simulink model "Example_Simulation"  (R2023b)
settings: Solver=FixedStepAuto  StartTime=0.0  StopTime=50  FixedStep=0.01  RelTol=1e-3
values from neighbouring files (symbols this model uses):
  A1 = [-1 x2min; 0 -1]    [Example_Code.m]
  A2 = [-1 x2max; 0 -1]    [Example_Code.m]
  B = [0 1].'    [Example_Code.m]
  x2max = 0.3    [Example_Code.m]
  x2min = 0.1    [Example_Code.m]
undefined symbols (not defined in the file or in its folder): adis1, adis2, bdis1, bdis2
libraries: simulink x1
settings Model: Creator=adria  LastModifiedBy=adria

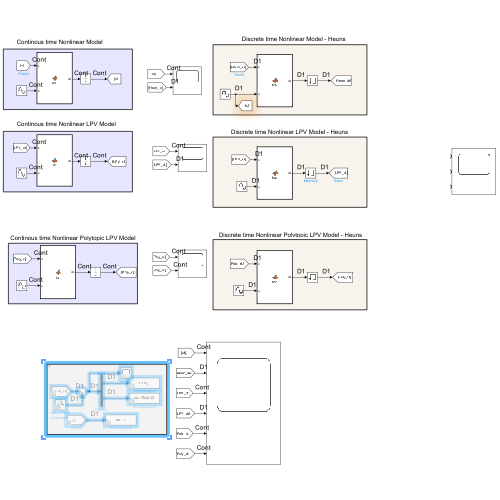
[thumbnail: Simulink's stored preview of the top-level diagram]
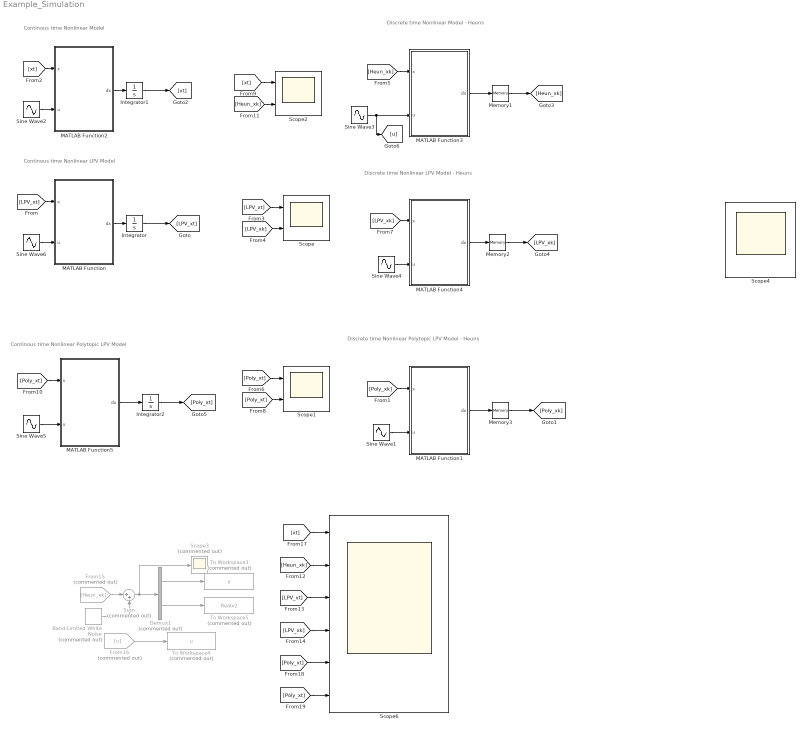
== system Example_Simulation ==
  note: Continous time Nonlinear LPV Model
  note: Continous time Nonlinear Model
  note: Discrete time Nonlinear Model - Heuns
  note: Discrete time Nonlinear LPV Model - Heuns
  note: Discrete time Nonlinear Polytopic LPV Model - Heuns
  note: Continous time Nonlinear Polytopic LPV Model
  Band-Limited White Noise : simulink/Sources/Band-Limited White Noise  Commented=on  Cov=[0.000001]  Ts=0.01  seed=[23341]
  Demux1 : Demux  Commented=on  Outputs=2
  From15 : From  Commented=on  GotoTag=Heun_xk
  From16 : From  Commented=on  GotoTag=u
  Integrator : Integrator  InitialCondition=[0 0.2].'
  Integrator1 : Integrator  InitialCondition=[0 0.2].'
  Integrator2 : Integrator  InitialCondition=[0 0.2].'
  MATLAB Function : MATLAB Function  TreatAsAtomicUnit=on
  MATLAB Function1 : MATLAB Function  TreatAsAtomicUnit=on
  MATLAB Function2 : MATLAB Function  TreatAsAtomicUnit=on
  MATLAB Function3 : MATLAB Function  TreatAsAtomicUnit=on
  MATLAB Function4 : MATLAB Function  TreatAsAtomicUnit=on
  MATLAB Function5 : MATLAB Function  TreatAsAtomicUnit=on
  Memory1 : Memory  InitialCondition=[0 0.2].'
  Memory2 : Memory  InitialCondition=[0 0.2].'
  Memory3 : Memory  InitialCondition=[0 0.2].'
  Scope : Scope  NumInputPorts=2
  Scope1 : Scope  NumInputPorts=2
  Scope2 : Scope  NumInputPorts=2
  Scope3 : Scope  Commented=on
  Scope4 : Scope  NumInputPorts=3
  Scope6 : Scope  NumInputPorts=6
  Sine Wave1 : Sin  Amplitude=0.1  Bias=0.2  Frequency=0.16  SampleTime=0.01
  Sine Wave2 : Sin  Amplitude=0.1  Bias=0.2  Frequency=0.16  SampleTime=0
  Sine Wave3 : Sin  Amplitude=0.1  Bias=0.2  Frequency=0.16  SampleTime=0.01
  Sine Wave4 : Sin  Amplitude=0.1  Bias=0.2  Frequency=0.16  SampleTime=0.01
  Sine Wave5 : Sin  Amplitude=0.1  Bias=0.2  Frequency=0.16  SampleTime=0
  Sine Wave6 : Sin  Amplitude=0.1  Bias=0.2  Frequency=0.16  SampleTime=0
  Sum : Sum  Commented=on  Inputs=|++
  To Workspace3 : ToWorkspace  Commented=on  VariableName=y  SaveFormat=Structure  SampleTime=-1
  To Workspace4 : ToWorkspace  Commented=on  VariableName=u  SaveFormat=Structure  SampleTime=-1
  To Workspace5 : ToWorkspace  Commented=on  VariableName=Realx2  SaveFormat=Structure  SampleTime=-1
  wires:
  MATLAB Function/1(dx) -> Integrator/1
  Integrator/1 -> [LPV_xt]
  Sine Wave6/1 -> MATLAB Function/2(u)
  [LPV_xt] -> MATLAB Function/1(x)
  [xt] -> MATLAB Function2/1(x)
  MATLAB Function2/1(dx) -> Integrator1/1
  Integrator1/1 -> [xt]
  Sine Wave2/1 -> MATLAB Function2/2(u)
  Memory1/1 -> [Heun_xk]
  Sine Wave3/1 -> [u], MATLAB Function3/2(u)
  [Heun_xk] -> MATLAB Function3/1(x)
  MATLAB Function3/1(dx) -> Memory1/1
  Sine Wave4/1 -> MATLAB Function4/2(u)
  MATLAB Function4/1(dx) -> Memory2/1
  [LPV_xk] -> MATLAB Function4/1(x)
  Memory2/1 -> [LPV_xk]
  Memory3/1 -> [Poly_xk]
  MATLAB Function1/1(dx) -> Memory3/1
  [Poly_xk] -> MATLAB Function1/1(x)
  Sine Wave1/1 -> MATLAB Function1/2(u)
  [Poly_xt] -> MATLAB Function5/1(x)
  Integrator2/1 -> [Poly_xt]
  MATLAB Function5/1(dx) -> Integrator2/1
  Sine Wave5/1 -> MATLAB Function5/2(u)
  [LPV_xt] -> Scope/1
  [LPV_xk] -> Scope/2
  [Poly_xt] -> Scope1/2
  [Poly_xt] -> Scope1/1
  [Heun_xk] -> Scope2/2
  [xt] -> Scope2/1
  [LPV_xk] -> Scope6/4
  [LPV_xt] -> Scope6/3
  [xt] -> Scope6/1
  [Heun_xk] -> Scope6/2
  [Poly_xt] -> Scope6/6
  [Poly_xt] -> Scope6/5
  Demux1/2 -> To Workspace5/1
  Demux1/1 -> To Workspace3/1
  From16/1 -> To Workspace4/1
  From15/1 -> Sum/1
  Band-Limited White Noise/1 -> Sum/2
  Sum/1 -> Scope3/1, Demux1/1

== matlab function Example_Simulation/MATLAB Function1 ==
  data: x input; u input; dx output; bdis1 parameter; adis2 parameter; adis1 parameter; bdis2 parameter; x2max parameter; x2min parameter
function dx  = fcn(x,u, bdis1, adis2, adis1, bdis2,x2max, x2min)


SchedulingMin = (x2max-x(2))/(x2max-x2min);
SchedulingMax = (1-SchedulingMin);

X = [x(1);x(2)];

dx = SchedulingMin*(adis1*X+bdis1*u) + SchedulingMax*(adis2*X+bdis2*u);

== matlab function Example_Simulation/MATLAB Function ==
  data: x input; dx output; u input
function dx = fcn(x,u)

X = [x(1);x(2)];
dx = [-1 x(2); 0 -1]*X+[0 1].'*u;

== matlab function Example_Simulation/MATLAB Function2 ==
  data: x input; dx output; u input
function dx = fcn(x,u)

dx1 = -x(1)+x(2)^2;
dx2 = -x(2)+u;
dx = [dx1;dx2];

== matlab function Example_Simulation/MATLAB Function3 ==
  data: x input; dx output; u input
function dx  = fcn(x,u)

dt = 0.01;
x1Predict = (-x(1)+x(2)^2)*dt+x(1);
x2Predict = (-x(2)+u)*dt+x(2);

T1 = -x(1)+x(2)^2;
N1 = -x1Predict+x2Predict^2;

T2 = -x(2)+u;
N2 = -x2Predict+u;

dx1 = x(1)+(dt/2)*(T1+N1);
dx2 = x(2)+(dt/2)*(T2+N2);

dx = [dx1;dx2];

== matlab function Example_Simulation/MATLAB Function4 ==
  data: x input; dx output; u input
function dx  = fcn(x,u)

dt = 0.01;


%% PREDICTED STATES
x1Predict = (-x(1)+x(2)^2)*dt+x(1);
x2Predict = (-x(2)+u)*dt+x(2);

%%  STATE VECTOR
X = [x(1);x(2)];

%%  PREDICTED STATE VECTOR
XPredict = [x1Predict;x2Predict];

%% DYNAMICS
Act1 = [-1 x(2); 0 -1]*X;
B1 = [0;1]*u;

%% PREDICTED DYNAMICS
Act2 = [-1 x2Predict; 0 -1]*XPredict;
B2 = [0;1]*u;

%% OUTPUT
dx = [x(1);x(2)]+(dt/2)*((Act1+Act2)+(B1+B2));

== matlab function Example_Simulation/MATLAB Function5 ==
  data: x input; u input; dx output; A1 parameter; A2 parameter; B parameter; x2max parameter; x2min parameter
function dx  = fcn(x,u, A1,A2,B,x2max, x2min)


SchedulingMin = (x2max-x(2))/(x2max-x2min);
SchedulingMax = (1-SchedulingMin);

X = [x(1);x(2)];

dx = SchedulingMin*(A1*X+B*u) + SchedulingMax*(A2*X+B*u);
